simulink library "lib_Convection_ColebrookCorr"  (R2015a)
settings: Solver=ode45  StartTime=0.0  StopTime=10.0  RelTol=1e-3
settings Model: Creator=jlkratz  LastModifiedBy=jlkratz

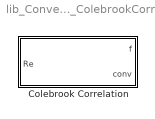
== system lib_Convection_ColebrookCorr ==
  Colebrook Correlation : Subsystem  mask(TSAT: Colebrook Correlation){eoD_M=0.02, BN_M=double(gcb)}
      mask prompts: eoD_M "eoD_M - Relative roughness: surface roughness divided by the hydraulic diameter of the pipe (e/D)"; BN_M "BN_M - Block Name"
      mask help: This block approximates the friction factor for fully developed flow in a pipe using the Colebrook correlation. The correlation accounts for surface roughness. The Colebrook correlation is solved in this block using the secant root method. The Reynolds number must be calculated using the hydraulic diamter of the pipe.
      mask Help: web(which('Convection_TSAT_ColebrookCorr.html'),'-helpbrowser')
      mask DialogControl Container4 Prompt: Parameters

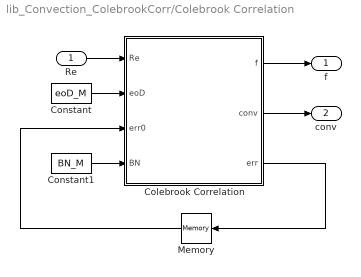
== system lib_Convection_ColebrookCorr/Colebrook Correlation ==
  Re : Inport
  Colebrook Correlation : MATLAB Function  TreatAsAtomicUnit=on
  Constant : Constant  Value=eoD_M
  Constant1 : Constant  Value=BN_M
  Memory : Memory  X0=zeros(1,7)
  f : Outport
  conv : Outport  Port=2
  wires:
  Constant/1 -> Colebrook Correlation/2(eoD)
  Colebrook Correlation/2(conv) -> conv/1
  Re/1 -> Colebrook Correlation/1(Re)
  Colebrook Correlation/1(f) -> f/1
  Constant1/1 -> Colebrook Correlation/4(BN)
  Colebrook Correlation/3(err) -> Memory/1
  Memory/1 -> Colebrook Correlation/3(err0)

== matlab function lib_Convection_ColebrookCorr/Colebrook Correlation/Colebrook Correlation ==
  data: Re input; f output; eoD input; conv output; err0 input; BN input; err output
function [f,conv,err] = ColebrookCorr(Re,eoD,err0,BN)
%#codegen

%Warning/Error Check
err = err0;
errNum = 1;
%Re is a 1-D array?
if min(size(Re)) ~= 1 && err0(errNum) ~= 1
    fprintf('warning in %s: Re must be a scalar or 1-D array\n',char(BN));
    err(errNum) = 1;
end
errNum = errNum + 1;
%eoD is a 1-D array?
if min(size(eoD)) ~= 1 && err0(errNum) ~= 1
    fprintf('warning in %s: eoD_M must be a scalar or 1-D array\n',char(BN));
    err(errNum) = 1;
end
errNum = errNum + 1;
%Re and eoD are the same size?
if length(Re) ~= length(eoD) && err0(errNum) ~= 1
    fprintf('warning in %s: Re and eoD_M must have the same number of elements\n',char(BN));
    err(errNum) = 1;
end
errNum = errNum + 1;
%Re has real positive elements?
if (min(isreal(Re)) ~= 1 || min(Re) < 0) && err0(errNum) ~= 1
    fprintf('warning in %s: Re must have all real positive elements\n',char(BN));
    err(errNum) = 1;
end
errNum = errNum + 1;
%eoD has real positive elements?
if (min(isreal(eoD)) ~= 1 || min(eoD) < 0) && err0(errNum) ~= 1
    fprintf('warning in %s: eoD_M must have all real positive elements\n',char(BN));
    err(errNum) = 1;
end
errNum = errNum + 1;
%Re has all finite elements?
if (max(isnan(Re)) > 0 || max(isinf(Re)) > 0) && err0(errNum) ~= 1
    fprintf('warning in %s: Re must have all finite elements\n',char(BN));
    err(errNum) = 1;
end
errNum = errNum + 1;
%eoD has all finite elements?
if (max(isnan(eoD)) > 0 || max(isinf(eoD)) > 0) && err0(errNum) ~= 1
    fprintf('warning in %s: eoD_M must have all finite elements\n',char(BN));
    err(errNum) = 1;
end

%Solve the Colebrook Correlation using the Secant Root Method
Xa = 0.02;
Xb = 0.04;
Err = 0.0001;
imax = 1000;

conv = ones(1,length(Re));
f = zeros(1,length(Re));
for j = 1:length(Re);
Xs = 0;
for i = 1:imax %Number iterations is specified by user
    FunXb = 1/sqrt(Xb) + 2*log10((eoD(j))/3.7 + 2.51/(Re(j)*sqrt(Xb))); %Value function at Xb is calculated
    FunXa = 1/sqrt(Xa) + 2*log10((eoD(j))/3.7 + 2.51/(Re(j)*sqrt(Xa))); %Value function at Xa is calculated
    Xi = Xb - FunXb*(Xa-Xb)/(FunXa-FunXb); %defines new solution by secant method
    %Avoid negative friction factor
    if Xi <= 0
        Xi = Xa/100;
    end
    if abs((Xi - Xb)/Xb) < Err %if error specification is met Xs is found and loop ends
        Xs = Xi;
        conv(j) = 1;
        break
    end
    Xa = Xb; %if error in solution is not met Xa become Xb
    Xb = Xi; %and Xb become Xi for next iteration
end
if i == imax %if an acceptable solution is not found in imax iteration, and error message is displayed
    conv(j) = 0;
    fprintf('Solution was not obtained in the specifed number of iterations.\n')
end
f(j) = Xs;
end
